simulink model "Tutorial3_Gazebo"  (Simulink 9.1)
settings: Solver=FixedStepAuto  StartTime=0.0  StopTime=10.0  FixedStep=0.01  RelTol=1e-3
libraries: WBToolboxLibrary x5
settings Model: SuppressorTable=22 serialization::archive 11 0 6 0 0 0 1 0  Creator=dferigo  LastModifiedBy=dferigo
settings DataIOCC: SaveFormat=Dataset
settings OptimizationCC: LifeSpan=auto
settings DebuggingCC: UnderspecifiedInitializationDetection=Simplified  MergeDetectMultiDrivingBlocksExec=error  SFUnexpectedBacktrackingDiag=error  SFNoUnconditionalDefaultTransitionDiag=error  SFExecutionAtInitializationDiag=warning
settings HardwareCC: ProdBitPerPointer=64  ProdBitPerSizeT=64  ProdBitPerPtrDiffT=64  ProdLargestAtomicFloat=Float  ProdIntDivRoundTo=Zero  ProdEndianess=LittleEndian  ProdWordSize=64  ProdHWDeviceType=Intel->x86-64 (Windows64)
settings ModelReferenceCC: PropagateSignalLabelsOutOfModel=on
settings CodeAppCC: StateflowObjectComments=off
settings GRTTargetCC: TargetLangStandard=C99 (ISO)  CombineOutputUpdateFcns=on  GRTInterface=off
settings ConfigComp: CovMetricSettings=dwe  CovHtmlReporting=off  CovSaveCumulativeToWorkspaceVar=off  CovSaveSingleToWorkspaceVar=off  CovExternalEMLEnable=on

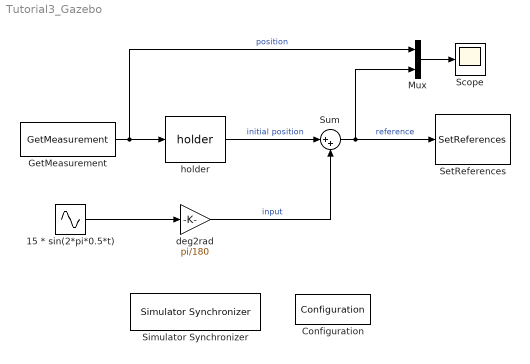
== system Tutorial3_Gazebo ==
  15 * sin(2*pi*0.5*t) : Sin  Amplitude=15  Frequency=2*pi*0.5  SampleTime=0
  Configuration : WBToolboxLibrary/Utilities/Configuration  ConfigSource=Mask  ConfigObject='WBTConfigRobot'  RobotName='icubSim'  UrdfFile='model.urdf'  ControlledJoints={'r_elbow'}  ControlBoardsNames={'right_arm'}  LocalName='WBT'  GravityVector=[0,0,-9.81]
      settings: SourceProductName=WholeBodyToolbox
  GetMeasurement : WBToolboxLibrary/States/GetMeasurement  measuredType=Joints Position
      settings: SourceProductName=WholeBodyToolbox
  Mux : Mux  Inputs=2
  Scope : Scope
  SetReferences : WBToolboxLibrary/Actuators/SetReferences  controlType=Position Direct  refSpeed=10*(pi/180)  refAcceleration=1000000*(pi/180)
      settings: SourceProductName=WholeBodyToolbox
  Simulator Synchronizer : WBToolboxLibrary/Utilities/Simulator Synchronizer  period=0.01  serverPortName='/clock/rpc'  clientPortName='/WBT_synchronizer/rpc:o'
      settings: SourceProductName=WholeBodyToolbox
  Sum : Sum  Inputs=|++
  deg2rad : Gain  Gain=pi/180
  "holder " : WBToolboxLibrary/Utilities/holder 
      settings: SourceProductName=WholeBodyToolbox
  wires:
  15 * sin(2*pi*0.5*t)/1 -> deg2rad/1
  GetMeasurement/1 -> Mux/1, "holder "/1  "position"
  "holder "/1 -> Sum/1  "initial position"
  deg2rad/1 -> Sum/2  "input"
  Sum/1 -> SetReferences/1, Mux/2  "reference"
  Mux/1 -> Scope/1
